simulink subsystem "Control"  (R2024a)
settings: Solver=VariableStepAuto  StartTime=0.0  StopTime=10.0  RelTol=1e-3
settings Model: Creator=gurt1  LastModifiedBy=gurt1
settings RTWCC: GPUComputeCapability=3.5

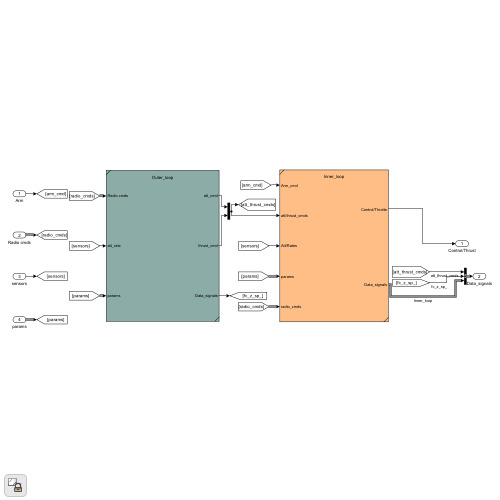
[thumbnail: Simulink's stored preview of the top-level diagram]
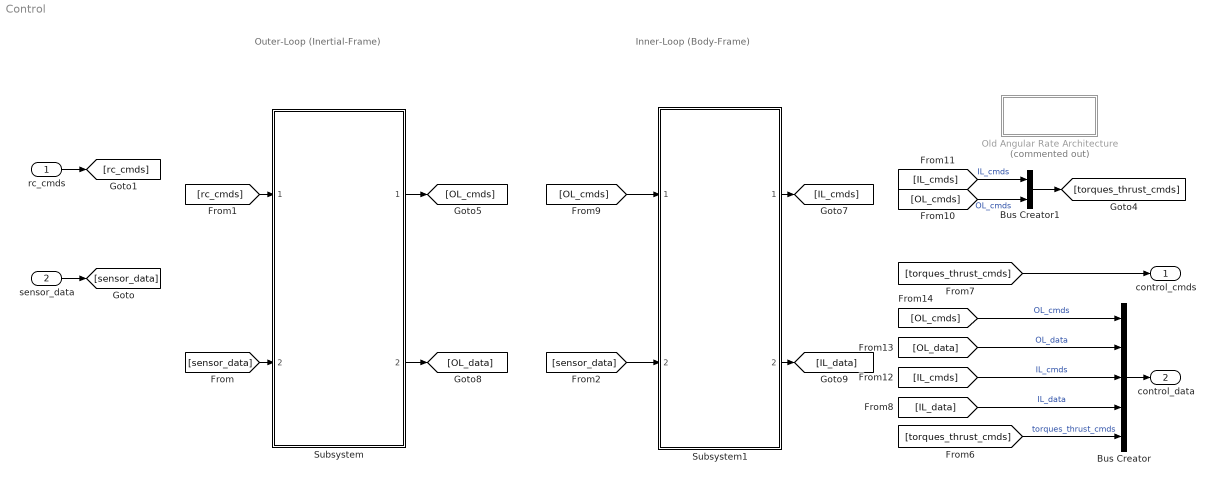
== system Control ==
  note: Inner-Loop (Body-Frame)
  note: Outer-Loop (Inertial-Frame)
  rc_cmds : Inport
  sensor_data : Inport  Port=2
  Bus Creator : BusCreator  Inputs=5
  Bus Creator1 : BusCreator  Inputs=2
  Old Angular Rate Architecture : Subsystem  Commented=on
  Subsystem : Subsystem  ReferencedSubsystem=Outer_loop
  Subsystem1 : Subsystem  ReferencedSubsystem=Inner_loop
  control_cmds : Outport
  control_data : Outport  Port=2
  wires:
  sensor_data/1 -> [sensor_data]
  [sensor_data] -> Subsystem/2
  rc_cmds/1 -> [rc_cmds]
  [rc_cmds] -> Subsystem/1
  [sensor_data] -> Subsystem1/2
  [torques_thrust_cmds] -> Bus Creator/5  "torques_thrust_cmds"
  Bus Creator/1 -> control_data/1
  Bus Creator1/1 -> [torques_thrust_cmds]
  Subsystem1/1 -> [IL_cmds]
  [OL_cmds] -> Subsystem1/1
  Subsystem1/2 -> [IL_data]
  [IL_data] -> Bus Creator/4  "IL_data"
  [torques_thrust_cmds] -> control_cmds/1
  [OL_data] -> Bus Creator/2  "OL_data"
  Subsystem/1 -> [OL_cmds]
  Subsystem/2 -> [OL_data]
  [OL_cmds] -> Bus Creator1/2  "OL_cmds"
  [IL_cmds] -> Bus Creator/3  "IL_cmds"
  [OL_cmds] -> Bus Creator/1  "OL_cmds"
  [IL_cmds] -> Bus Creator1/1  "IL_cmds"

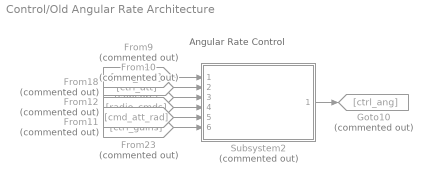
== system Control/Old Angular Rate Architecture ==
  note: Angular Rate Control
  From10 : From  Commented=on  GotoTag=sensors
  From11 : From  Commented=on  GotoTag=ctrl_gains
  From12 : From  Commented=on  GotoTag=radio_cmds
  From18 : From  Commented=on  GotoTag=ctrl_att
  From23 : From  Commented=on  GotoTag=cmd_att_rad
  From9 : From  Commented=on  GotoTag=arm_cmd
  Goto10 : Goto  Commented=on  GotoTag=ctrl_ang
  Subsystem2 : Subsystem  Commented=on  ReferencedSubsystem=Angular_Rate
  wires:
  From10/1 -> Subsystem2/3
  Subsystem2/1 -> Goto10/1
  From12/1 -> Subsystem2/4
  From23/1 -> Subsystem2/5
  From9/1 -> Subsystem2/1
  From11/1 -> Subsystem2/6
  From18/1 -> Subsystem2/2
